simulink library "ECI2OEV_lib"  (R2016b)
settings: Solver=VariableStepAuto  StartTime=0.0  StopTime=10.0  RelTol=1e-3
settings Model: Creator=Taylor  LastModifiedBy=taylorreynolds

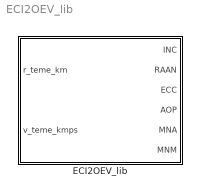
== system ECI2OEV_lib ==
  ECI2OEV_lib : Subsystem

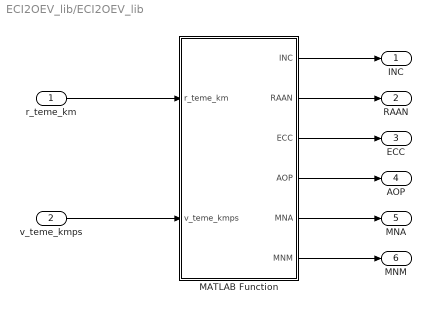
== system ECI2OEV_lib/ECI2OEV_lib ==
  r_teme_km : Inport
  v_teme_kmps : Inport  Port=2
  MATLAB Function : MATLAB Function  TreatAsAtomicUnit=on
  INC : Outport
  RAAN : Outport  Port=2
  ECC : Outport  Port=3
  AOP : Outport  Port=4
  MNA : Outport  Port=5
  MNM : Outport  Port=6
  wires:
  MATLAB Function/1(INC) -> INC/1
  MATLAB Function/2(RAAN) -> RAAN/1
  MATLAB Function/3(ECC) -> ECC/1
  MATLAB Function/4(AOP) -> AOP/1
  MATLAB Function/5(MNA) -> MNA/1
  MATLAB Function/6(MNM) -> MNM/1
  v_teme_kmps/1 -> MATLAB Function/2(v_teme_kmps)
  r_teme_km/1 -> MATLAB Function/1(r_teme_km)

== matlab function ECI2OEV_lib/MATLAB Function ==
  data: r_teme_km input size=3; INC output size=1; v_teme_kmps input size=3; RAAN output size=1; ECC output size=1; AOP output size=1; MNA output size=1; MNM output size=1
function [INC,RAAN,ECC,AOP,MNA,MNM] = ECI2OEV(r_teme_km,v_teme_kmps)
% Converts ECI position and velocity to classical orbital elements.
%   UW HuskySat-1, ADCS Subsystem
%   Updated: T. Reynolds 12.15.17
% #codegen

% Input

%  r_eci_m = eci position vector [meters]
%  v_eci_mps = eci velocity vector [meters/second]

% Output

% INC   = orbital inclination [degrees]
% RAAN  = right ascension of ascending node [degrees]
% ECC   = orbital eccentricity [-]
% AOP   = argument of perigee [degrees]
% MNA   = mean anomaly [degrees]
% MNM   = mean motion [orbits/day]

% Reference: Spacecraft Dynamics and Control, M. Sidi. Vallado, 2014.

% ----- Constants ----- %
mu          = 398600.4418;      % km3/s2
small       = 1.0e-10;
twopi       = 2.0 * pi;
halfpi      = 0.5 * pi;
sinday      = 24 * 3600;
rad         = 180.0 / pi;
sqrt_mu     = sqrt(mu);
pi2 = pi*pi;
r   = r_teme_km;
v   = v_teme_kmps;

% -------------------------  implementation   -----------------
MNA     = 0.0;
magr = norm( r );
magv = norm( v );
% ------------------  find h n and e vectors   ----------------
hbar    = cross( r,v );
magh    = norm( hbar );
nbar    = [ -hbar(2); hbar(1); 0.0 ];
magn    = norm( nbar );
c1      = magv*magv - mu /magr;
rdotv   = dot( r,v );

ebar    = zeros(3,1);
for i = 1:3
    ebar(i)= (c1*r(i) - rdotv*v(i))/mu;
end
ECC = norm( ebar );

% ------------  find a e and semi-latus rectum   ----------
sme     = ( magv*magv*0.5  ) - ( mu /magr );
%if ( abs( sme ) > small )
    a   = -mu  / (2.0 *sme);
% else
%     a   = infinite;
% end
% p   = magh*magh/mu;

% -------------------  find mean motion   -----------------
MNM     = sqrt(mu/a^3);
MNM     = MNM/(twopi/sinday);

 % -----------------  find inclination   -------------------
hk    = hbar(3)/magh;
INC   = acos( hk );

% --------  determine type of orbit for later use  --------
% ------ elliptical, parabolic, hyperbolic inclined -------
typeorbit= 'ei';
if ( ECC < small )
    % ----------------  circular equatorial ---------------
    if  (INC<small) || (abs(INC-pi)<small)
        typeorbit= 'ce';
    else
        % --------------  circular inclined ---------------
        typeorbit= 'ci';
    end
else
    % - elliptical, parabolic, hyperbolic equatorial --
    if  (INC<small) || (abs(INC-pi)<small)
        typeorbit= 'ee';
    end
end

% ----------  find longitude of ascending node ------------
%if ( magn > small )
    temp = nbar(1) / magn;
    if ( abs(temp) > 1.0  )
        temp = sign(temp);
    end
    RAAN = acos( temp );
    if ( nbar(2) < 0.0  )
        RAAN = twopi - RAAN;
    end
% else
%     omega = undefined;
% end

% ---------------- find argument of perigee ---------------
if( strcmp(typeorbit,'ei') == 1 )
    AOP = angl( nbar,ebar);
    if ( ebar(3) < 0.0  )
        AOP = twopi - AOP;
    end
else
    AOP = inf;
end


% ------------  find true anomaly at epoch    -------------
if ( typeorbit(1:1) == 'e' )
    nu =  angl( ebar,r );
    if ( rdotv < 0.0  )
        nu = twopi - nu;
    end
else
    nu = inf;
end

% ----  find argument of latitude - circular inclined -----
if (strcmp(typeorbit, 'ci') == 1)
    arglat = angl( nbar,r );
    if ( r(3) < 0.0  )
        arglat= twopi - arglat;
    end
    MNA = arglat;
end

% -- find longitude of perigee - elliptical equatorial ----
% if  ( ECC>small ) && (strcmp(typeorbit, 'ee') == 1)
%     temp = ebar(1)/ECC;
%     if ( abs(temp) > 1.0  )
%         temp = sign(temp);
%     end
%     lonper = acos( temp );
%     if ( ebar(2) < 0.0  )
%         lonper = twopi - lonper;
%     end
%     if ( INC > halfpi )
%         lonper = twopi - lonper;
%     end
% else
%     lonper = inf;
% end

% -------- find true longitude - circular equatorial ------
if(strcmp(typeorbit, 'ce') == 1)
    temp = r(1)/magr;
    if ( abs(temp) > 1.0  )
        temp = sign(temp);
    end
    truelon = acos( temp );
    if ( r(2) < 0.0  )
        truelon = twopi - truelon;
    end
    if ( INC > halfpi )
        truelon = twopi - truelon;
    end
    MNA = mod(truelon - AOP,twopi);
end

% ------------ find mean anomaly for all orbits -----------
if ( typeorbit(1:1) == 'e' )
    [~,MNA] = newtonnu(ECC,nu );
end

INC     = rad*INC;
RAAN    = rad*RAAN;
AOP     = rad*AOP;
MNA     = rad*MNA;

% % negative orbital energy
% noe     = mu/r - 0.5*v*v;
% 
% % compute semi-major axis
% a   = 0.5*mu/noe;
% a3  = a*a*a;
% 
% % compute orbital angular momentum
% H   = cross(r_eci_m,v_eci_mps);
% hx  = H(1);
% hy  = H(2);
% hz  = H(3);
% h   = norm(H);
% hxy     = sqrt(hx^2 + hy^2);
% 
% % compute inclination
% INC = acosd(hz/h);
% 
% % compute right ascension of ascending node in the correct quadrant
% sOm     = hx/hxy;
% cOm     = -hy/hxy;
% RAAN     = getQuadrant(cOm,sOm);
%     
% % compute eccentricity
% ECC   = sqrt( 1 - h^2/(mu*a) );
% 
% % compute eccentric anomaly
% cE  = (a - r)/(a*ECC);
% sE  = dot(r,v)/(ECC*sqrt(mu*a));
% E   = getQuadrant(cE,sE);
% 
% % compute true anomaly
% cth     = (cE-ECC)/(1-ECC*cE);
% sth     = (sE*(sqrt(1-ECC^2))/(1 - ECC*cE));
% TRA     = getQuadrant(cth,sth);
% 
% % compute mean anomaly
% MNA     = E - ECC*sE;
% 
% % compute argument of perigee
% s_wpth      = z/(r*sind(INC));
% c_wpth      = (x*cosd(RAAN) + y*sind(RAAN))/r;
% wpth        = getQuadrant(c_wpth,s_wpth);
% AOP         = wpth - TRA;
% 
% % compute mean motion
% MNM     = sqrt_mu/a3; % [rad/s]
% MNM     = MNM/(pi2/1440.0); % [orbit/day]

end

% function angle = getQuadrant(cAngle,sAngle)
% 
% anglec  = acosd(cAngle);
% 
% if( cAngle < 0 )
%     if( sAngle < 0 )
%         angle = anglec + 90; % third quadrant
%     else
%         angle = anglec; % second quadrant
%     end
% else
%     if( sOm < 0 )
%         angle = 360 - anglec; % fourth quadrant
%     else
%         angle = anglec; % first quadrant
%     end
% end
% 
% end

function theta = angl ( vec1,vec2 )
small     = 0.00000001;
undefined = 999999.1;

magv1 = norm(vec1);
magv2 = norm(vec2);

if( magv1*magv2 > small^2 )
    temp = dot(vec1,vec2) / (magv1*magv2);
    if abs( temp ) > 1.0
        temp = sign(temp) * 1.0;
    end
    theta = acos( temp );
else
    theta = undefined;
end
end

function [e0,m] = newtonnu ( ecc,nu )

% ---------------------  implementation   ---------------------
e0= 999999.9;
m = 999999.9;
small = 0.00000001;

% --------------------------- circular ------------------------
if ( abs( ecc ) < small  )
    m = nu;
    e0= nu;
else
    % ---------------------- elliptical -----------------------
    if ( ecc < 1.0-small  )
        sine= ( sqrt( 1.0 -ecc*ecc ) * sin(nu) ) / ( 1.0 +ecc*cos(nu) );
        cose= ( ecc + cos(nu) ) / ( 1.0  + ecc*cos(nu) );
        e0  = atan2( sine,cose );
        m   = e0 - ecc*sin(e0);
    else
        % -------------------- hyperbolic  --------------------
        if ( ecc > 1.0 + small  )
            if (ecc > 1.0 ) && (abs(nu)+0.00001 < pi-acos(1.0 /ecc))
                sine= ( sqrt( ecc*ecc-1.0  ) * sin(nu) ) / ( 1.0  + ecc*cos(nu) );
                e0  = asinh( sine );
                m   = ecc*sinh(e0) - e0;
            end
        else
            % ----------------- parabolic ---------------------
            if ( abs(nu) < 168.0*pi/180.0  )
                e0= tan( nu*0.5  );
                m = e0 + (e0*e0*e0)/3.0;
            end
        end
    end
end

if ( ecc < 1.0  )
    m = rem( m,2.0 *pi );
    if ( m < 0.0  )
        m= m + 2.0 *pi;
    end
    e0 = rem( e0,2.0 *pi );
end

end
